simulink model "mini_project_2"  (R2024b)
settings: Solver=VariableStepAuto  StartTime=0.0  StopTime=10.0  RelTol=1e-3
values from neighbouring files (symbols this model uses):
  g = 9.81    [mini_project_2_par.m]    (also in mini_project_par.m = 9.82)
  Ic = diag([ 2 ; 2 ; 4 ])    [mini_project_2_par.m]
  m = 4    [mini_project_2_par.m]    (also in mini_project_par.m = 0.725)
  M_RB = [ m*eye(3) , zeros(3) ; zeros(3) , Ic ]    [mini_project_2_par.m]
  omega_pars = [omega_min, omega_max]    [mini_project_par.m]
  params = [m, g, h L, Ct, Ixx, Iyy, Izz]    [mini_project_par.m]
libraries: slpidlib x12, simulink_extras x7, aerolibutil x2, vrlib x1
(part 2 of 2)

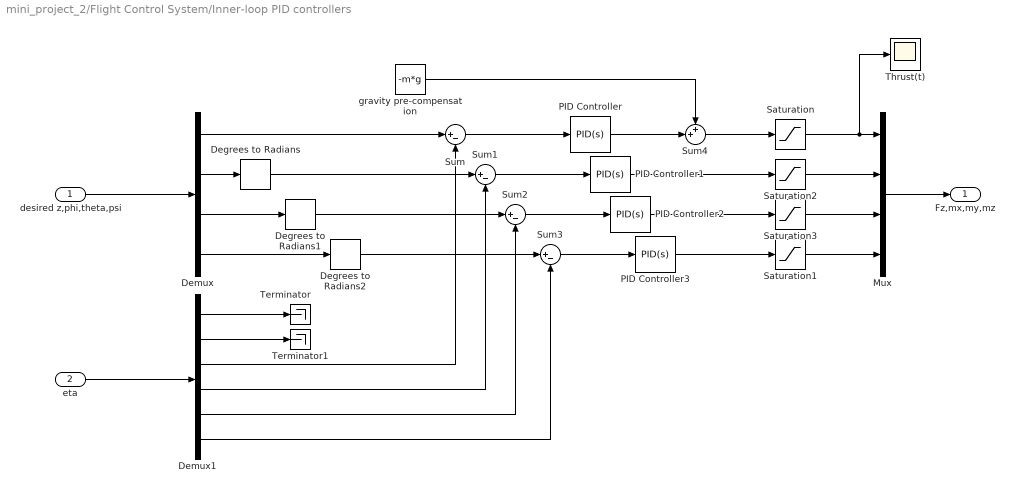
== system mini_project_2/Flight Control System/Inner-loop PID controllers ==
  desired z,phi,theta,psi : Inport
  eta : Inport  Port=2
  Degrees to Radians : simulink_extras/Transformations/Degrees to Radians
  Degrees to Radians1 : simulink_extras/Transformations/Degrees to Radians
  Degrees to Radians2 : simulink_extras/Transformations/Degrees to Radians
  Demux : Demux
  Demux1 : Demux  Outputs=6
  Mux : Mux
  PID Controller : slpidlib/PID Controller  Controller=PID  Form=Parallel  TimeDomain=Continuous-time  UseExternalTs=off  SampleTime=-1  IntegratorMethod=Forward Euler  FilterMethod=Forward Euler  ControllerParametersSource=internal  P=10  I=0  UseKiTs=off  D=20  UseExternalDerivativeSource=off  N=110  UseFilter=on  TunerSelectOption=Transfer Function Based (PID Tuner App)  InitialConditionSource=internal  InitialConditionForIntegrator=0  InitialConditionForFilter=0  DifferentiatorICPrevScaledInput=0  ExternalReset=none  TrackingMode=off  Kt=1  LimitOutput=off  SatLimitsSource=internal  UpperSaturationLimit=100  LowerSaturationLimit=-100  LinearizeAsGain=on  AntiWindupMode=none  Kb=1  LimitIntegrator=off  UpperIntegratorSaturationLimit=inf  LowerIntegratorSaturationLimit=-inf  POutMin=[]  POutMax=[]  IOutMin=[]  IOutMax=[]  DOutMin=[]  DOutMax=[]  NOutMin=[]  NOutMax=[]  SumOutMin=[]  SumOutMax=[]  SaturationOutMin=[]  SaturationOutMax=[]  PParamMin=[]  PParamMax=[]  IParamMin=[]  IParamMax=[]  DParamMin=[]  DParamMax=[]  NParamMin=[]  NParamMax=[]  KbParamMin=[]  KbParamMax=[]  KtParamMin=[]  KtParamMax=[]  KbOutMin=[]  KbOutMax=[]  KtOutMin=[]  KtOutMax=[]  IntegratorOutMin=[]  IntegratorOutMax=[]  FilterOutMin=[]  FilterOutMax=[]  SumI1OutMin=[]  SumI1OutMax=[]  SumI2OutMin=[]  SumI2OutMax=[]  SumI3OutMin=[]  SumI3OutMax=[]  SumI4OutMin=[]  SumI4OutMax=[]  SumDOutMin=[]  SumDOutMax=[]  DifferentiatorOutMin=[]  DifferentiatorOutMax=[]  FilterDiffOutCoefMin=[]  FilterDiffOutCoefMax=[]  ReciprocalOutMin=[]  ReciprocalOutMax=[]  SumDenOutMin=[]  SumDenOutMax=[]  SumNumOutMin=[]  SumNumOutMax=[]  DivideOutMin=[]  DivideOutMax=[]  UdiffTsProdOutMin=[]  UdiffTsProdOutMax=[]  NTsProdOutMin=[]  NTsProdOutMax=[]  UintegralTsProdOutMin=[]  UintegralTsProdOutMax=[]  UngainTsProdOutMin=[]  UngainTsProdOutMax=[]  ClampingZeroOutDataTypeStr=Inherit: Inherit via back propagation  ClampingZeroOutMin=[]  ClampingZeroOutMax=[]  FilterDenConstantOutDataTypeStr=Inherit: Inherit via back propagation  FilterDenConstantOutMin=[]  FilterDenConstantOutMax=[]  PCopyOutDataTypeStr=Inherit: Inherit via back propagation  PCopyOutMin=[]  PCopyOutMax=[]  NCopyOutDataTypeStr=Inherit: Inherit via back propagation  NCopyOutMin=[]  NCopyOutMax=[]  IntegratorContinuousStateAttributes=''  IntegratorStateMustResolveToSignalObject=off  IntegratorRTWStateStorageClass=Auto  FilterContinuousStateAttributes=''  FilterStateMustResolveToSignalObject=off  FilterRTWStateStorageClass=Auto  ParallelPVariant=InternalParameters  IdealPVariant=Disabled  IVariant=InternalParameters  DVariant=InternalParameters  IntegratorVariant=Continuous  SatVariant=Disabled  AWVariant=Passthrough  PCopyVariant=Disabled  TRVariant=Disabled  FdbkBlocksVariant=Forward  IdealPFdbkVariant=Disabled  SatFdbkVariant=Disabled  DerivativeFilterVariant=ContFilter  NVariant=InternalParameters  NCopyVariant=Disabled  FilterICVariant=InternalICsFilter  IntegratorICVariant=InternalICs  ExternalResetVariant=Disabled  TRSumVariant=Passthrough  SumFdbkVariant=Disabled  SumVariant=Sum_PID  TsampFilterVariant=InternalTs  TsampNgainVariant=Passthrough  TsampIntegralVariant=Disabled_SignalSpec  ExternalSaturationOutDataTypeStr=Inherit: Same as second input  DerivativeSourceVariant=ErrorSignal  PreIntVariant=InternalPreInt
  PID Controller1 : slpidlib/PID Controller  Controller=PID  Form=Parallel  TimeDomain=Continuous-time  UseExternalTs=off  SampleTime=-1  IntegratorMethod=Forward Euler  FilterMethod=Forward Euler  ControllerParametersSource=internal  P=10  I=0  UseKiTs=off  D=20  UseExternalDerivativeSource=off  N=100  UseFilter=on  TunerSelectOption=Transfer Function Based (PID Tuner App)  InitialConditionSource=internal  InitialConditionForIntegrator=0  InitialConditionForFilter=0  DifferentiatorICPrevScaledInput=0  ExternalReset=none  TrackingMode=off  Kt=1  LimitOutput=off  SatLimitsSource=internal  UpperSaturationLimit=inf  LowerSaturationLimit=-inf  LinearizeAsGain=on  AntiWindupMode=none  Kb=1  LimitIntegrator=off  UpperIntegratorSaturationLimit=inf  LowerIntegratorSaturationLimit=-inf  POutMin=[]  POutMax=[]  IOutMin=[]  IOutMax=[]  DOutMin=[]  DOutMax=[]  NOutMin=[]  NOutMax=[]  SumOutMin=[]  SumOutMax=[]  SaturationOutMin=[]  SaturationOutMax=[]  PParamMin=[]  PParamMax=[]  IParamMin=[]  IParamMax=[]  DParamMin=[]  DParamMax=[]  NParamMin=[]  NParamMax=[]  KbParamMin=[]  KbParamMax=[]  KtParamMin=[]  KtParamMax=[]  KbOutMin=[]  KbOutMax=[]  KtOutMin=[]  KtOutMax=[]  IntegratorOutMin=[]  IntegratorOutMax=[]  FilterOutMin=[]  FilterOutMax=[]  SumI1OutMin=[]  SumI1OutMax=[]  SumI2OutMin=[]  SumI2OutMax=[]  SumI3OutMin=[]  SumI3OutMax=[]  SumI4OutMin=[]  SumI4OutMax=[]  SumDOutMin=[]  SumDOutMax=[]  DifferentiatorOutMin=[]  DifferentiatorOutMax=[]  FilterDiffOutCoefMin=[]  FilterDiffOutCoefMax=[]  ReciprocalOutMin=[]  ReciprocalOutMax=[]  SumDenOutMin=[]  SumDenOutMax=[]  SumNumOutMin=[]  SumNumOutMax=[]  DivideOutMin=[]  DivideOutMax=[]  UdiffTsProdOutMin=[]  UdiffTsProdOutMax=[]  NTsProdOutMin=[]  NTsProdOutMax=[]  UintegralTsProdOutMin=[]  UintegralTsProdOutMax=[]  UngainTsProdOutMin=[]  UngainTsProdOutMax=[]  ClampingZeroOutDataTypeStr=Inherit: Inherit via back propagation  ClampingZeroOutMin=[]  ClampingZeroOutMax=[]  FilterDenConstantOutDataTypeStr=Inherit: Inherit via back propagation  FilterDenConstantOutMin=[]  FilterDenConstantOutMax=[]  PCopyOutDataTypeStr=Inherit: Inherit via back propagation  PCopyOutMin=[]  PCopyOutMax=[]  NCopyOutDataTypeStr=Inherit: Inherit via back propagation  NCopyOutMin=[]  NCopyOutMax=[]  IntegratorContinuousStateAttributes=''  IntegratorStateMustResolveToSignalObject=off  IntegratorRTWStateStorageClass=Auto  FilterContinuousStateAttributes=''  FilterStateMustResolveToSignalObject=off  FilterRTWStateStorageClass=Auto  ParallelPVariant=InternalParameters  IdealPVariant=Disabled  IVariant=InternalParameters  DVariant=InternalParameters  IntegratorVariant=Continuous  SatVariant=Disabled  AWVariant=Passthrough  PCopyVariant=Disabled  TRVariant=Disabled  FdbkBlocksVariant=Forward  IdealPFdbkVariant=Disabled  SatFdbkVariant=Disabled  DerivativeFilterVariant=ContFilter  NVariant=InternalParameters  NCopyVariant=Disabled  FilterICVariant=InternalICsFilter  IntegratorICVariant=InternalICs  ExternalResetVariant=Disabled  TRSumVariant=Passthrough  SumFdbkVariant=Disabled  SumVariant=Sum_PID  TsampFilterVariant=InternalTs  TsampNgainVariant=Passthrough  TsampIntegralVariant=Disabled_SignalSpec  ExternalSaturationOutDataTypeStr=Inherit: Same as second input  DerivativeSourceVariant=ErrorSignal  PreIntVariant=InternalPreInt
  PID Controller2 : slpidlib/PID Controller  Controller=PID  Form=Parallel  TimeDomain=Continuous-time  UseExternalTs=off  SampleTime=-1  IntegratorMethod=Forward Euler  FilterMethod=Forward Euler  ControllerParametersSource=internal  P=10  I=0  UseKiTs=off  D=20  UseExternalDerivativeSource=off  N=100  UseFilter=on  TunerSelectOption=Transfer Function Based (PID Tuner App)  InitialConditionSource=internal  InitialConditionForIntegrator=0  InitialConditionForFilter=0  DifferentiatorICPrevScaledInput=0  ExternalReset=none  TrackingMode=off  Kt=1  LimitOutput=off  SatLimitsSource=internal  UpperSaturationLimit=inf  LowerSaturationLimit=-inf  LinearizeAsGain=on  AntiWindupMode=none  Kb=1  LimitIntegrator=off  UpperIntegratorSaturationLimit=inf  LowerIntegratorSaturationLimit=-inf  POutMin=[]  POutMax=[]  IOutMin=[]  IOutMax=[]  DOutMin=[]  DOutMax=[]  NOutMin=[]  NOutMax=[]  SumOutMin=[]  SumOutMax=[]  SaturationOutMin=[]  SaturationOutMax=[]  PParamMin=[]  PParamMax=[]  IParamMin=[]  IParamMax=[]  DParamMin=[]  DParamMax=[]  NParamMin=[]  NParamMax=[]  KbParamMin=[]  KbParamMax=[]  KtParamMin=[]  KtParamMax=[]  KbOutMin=[]  KbOutMax=[]  KtOutMin=[]  KtOutMax=[]  IntegratorOutMin=[]  IntegratorOutMax=[]  FilterOutMin=[]  FilterOutMax=[]  SumI1OutMin=[]  SumI1OutMax=[]  SumI2OutMin=[]  SumI2OutMax=[]  SumI3OutMin=[]  SumI3OutMax=[]  SumI4OutMin=[]  SumI4OutMax=[]  SumDOutMin=[]  SumDOutMax=[]  DifferentiatorOutMin=[]  DifferentiatorOutMax=[]  FilterDiffOutCoefMin=[]  FilterDiffOutCoefMax=[]  ReciprocalOutMin=[]  ReciprocalOutMax=[]  SumDenOutMin=[]  SumDenOutMax=[]  SumNumOutMin=[]  SumNumOutMax=[]  DivideOutMin=[]  DivideOutMax=[]  UdiffTsProdOutMin=[]  UdiffTsProdOutMax=[]  NTsProdOutMin=[]  NTsProdOutMax=[]  UintegralTsProdOutMin=[]  UintegralTsProdOutMax=[]  UngainTsProdOutMin=[]  UngainTsProdOutMax=[]  ClampingZeroOutDataTypeStr=Inherit: Inherit via back propagation  ClampingZeroOutMin=[]  ClampingZeroOutMax=[]  FilterDenConstantOutDataTypeStr=Inherit: Inherit via back propagation  FilterDenConstantOutMin=[]  FilterDenConstantOutMax=[]  PCopyOutDataTypeStr=Inherit: Inherit via back propagation  PCopyOutMin=[]  PCopyOutMax=[]  NCopyOutDataTypeStr=Inherit: Inherit via back propagation  NCopyOutMin=[]  NCopyOutMax=[]  IntegratorContinuousStateAttributes=''  IntegratorStateMustResolveToSignalObject=off  IntegratorRTWStateStorageClass=Auto  FilterContinuousStateAttributes=''  FilterStateMustResolveToSignalObject=off  FilterRTWStateStorageClass=Auto  ParallelPVariant=InternalParameters  IdealPVariant=Disabled  IVariant=InternalParameters  DVariant=InternalParameters  IntegratorVariant=Continuous  SatVariant=Disabled  AWVariant=Passthrough  PCopyVariant=Disabled  TRVariant=Disabled  FdbkBlocksVariant=Forward  IdealPFdbkVariant=Disabled  SatFdbkVariant=Disabled  DerivativeFilterVariant=ContFilter  NVariant=InternalParameters  NCopyVariant=Disabled  FilterICVariant=InternalICsFilter  IntegratorICVariant=InternalICs  ExternalResetVariant=Disabled  TRSumVariant=Passthrough  SumFdbkVariant=Disabled  SumVariant=Sum_PID  TsampFilterVariant=InternalTs  TsampNgainVariant=Passthrough  TsampIntegralVariant=Disabled_SignalSpec  ExternalSaturationOutDataTypeStr=Inherit: Same as second input  DerivativeSourceVariant=ErrorSignal  PreIntVariant=InternalPreInt
  PID Controller3 : slpidlib/PID Controller  Controller=PID  Form=Parallel  TimeDomain=Continuous-time  UseExternalTs=off  SampleTime=-1  IntegratorMethod=Forward Euler  FilterMethod=Forward Euler  ControllerParametersSource=internal  P=10  I=0  UseKiTs=off  D=20  UseExternalDerivativeSource=off  N=100  UseFilter=on  TunerSelectOption=Transfer Function Based (PID Tuner App)  InitialConditionSource=internal  InitialConditionForIntegrator=0  InitialConditionForFilter=0  DifferentiatorICPrevScaledInput=0  ExternalReset=none  TrackingMode=off  Kt=1  LimitOutput=off  SatLimitsSource=internal  UpperSaturationLimit=inf  LowerSaturationLimit=-inf  LinearizeAsGain=on  AntiWindupMode=none  Kb=1  LimitIntegrator=off  UpperIntegratorSaturationLimit=inf  LowerIntegratorSaturationLimit=-inf  POutMin=[]  POutMax=[]  IOutMin=[]  IOutMax=[]  DOutMin=[]  DOutMax=[]  NOutMin=[]  NOutMax=[]  SumOutMin=[]  SumOutMax=[]  SaturationOutMin=[]  SaturationOutMax=[]  PParamMin=[]  PParamMax=[]  IParamMin=[]  IParamMax=[]  DParamMin=[]  DParamMax=[]  NParamMin=[]  NParamMax=[]  KbParamMin=[]  KbParamMax=[]  KtParamMin=[]  KtParamMax=[]  KbOutMin=[]  KbOutMax=[]  KtOutMin=[]  KtOutMax=[]  IntegratorOutMin=[]  IntegratorOutMax=[]  FilterOutMin=[]  FilterOutMax=[]  SumI1OutMin=[]  SumI1OutMax=[]  SumI2OutMin=[]  SumI2OutMax=[]  SumI3OutMin=[]  SumI3OutMax=[]  SumI4OutMin=[]  SumI4OutMax=[]  SumDOutMin=[]  SumDOutMax=[]  DifferentiatorOutMin=[]  DifferentiatorOutMax=[]  FilterDiffOutCoefMin=[]  FilterDiffOutCoefMax=[]  ReciprocalOutMin=[]  ReciprocalOutMax=[]  SumDenOutMin=[]  SumDenOutMax=[]  SumNumOutMin=[]  SumNumOutMax=[]  DivideOutMin=[]  DivideOutMax=[]  UdiffTsProdOutMin=[]  UdiffTsProdOutMax=[]  NTsProdOutMin=[]  NTsProdOutMax=[]  UintegralTsProdOutMin=[]  UintegralTsProdOutMax=[]  UngainTsProdOutMin=[]  UngainTsProdOutMax=[]  ClampingZeroOutDataTypeStr=Inherit: Inherit via back propagation  ClampingZeroOutMin=[]  ClampingZeroOutMax=[]  FilterDenConstantOutDataTypeStr=Inherit: Inherit via back propagation  FilterDenConstantOutMin=[]  FilterDenConstantOutMax=[]  PCopyOutDataTypeStr=Inherit: Inherit via back propagation  PCopyOutMin=[]  PCopyOutMax=[]  NCopyOutDataTypeStr=Inherit: Inherit via back propagation  NCopyOutMin=[]  NCopyOutMax=[]  IntegratorContinuousStateAttributes=''  IntegratorStateMustResolveToSignalObject=off  IntegratorRTWStateStorageClass=Auto  FilterContinuousStateAttributes=''  FilterStateMustResolveToSignalObject=off  FilterRTWStateStorageClass=Auto  ParallelPVariant=InternalParameters  IdealPVariant=Disabled  IVariant=InternalParameters  DVariant=InternalParameters  IntegratorVariant=Continuous  SatVariant=Disabled  AWVariant=Passthrough  PCopyVariant=Disabled  TRVariant=Disabled  FdbkBlocksVariant=Forward  IdealPFdbkVariant=Disabled  SatFdbkVariant=Disabled  DerivativeFilterVariant=ContFilter  NVariant=InternalParameters  NCopyVariant=Disabled  FilterICVariant=InternalICsFilter  IntegratorICVariant=InternalICs  ExternalResetVariant=Disabled  TRSumVariant=Passthrough  SumFdbkVariant=Disabled  SumVariant=Sum_PID  TsampFilterVariant=InternalTs  TsampNgainVariant=Passthrough  TsampIntegralVariant=Disabled_SignalSpec  ExternalSaturationOutDataTypeStr=Inherit: Same as second input  DerivativeSourceVariant=ErrorSignal  PreIntVariant=InternalPreInt
  Saturation{,1..3} (4 alike) : Saturate  UpperLimit=100  LowerLimit=-100
  Sum{,1..3} (4 alike) : Sum  Inputs=|+-
  Sum4 : Sum  Inputs=++|
  Terminator : Terminator
  Terminator1 : Terminator
  Thrust(t) : Scope
  gravity pre-compensation : Constant  Value=-m*g
  Fz,mx,my,mz : Outport
  wires:
  Mux/1 -> Fz,mx,my,mz/1
  Sum/1 -> PID Controller/1
  Sum1/1 -> PID Controller1/1
  PID Controller1/1 -> Saturation2/1
  PID Controller2/1 -> Saturation3/1
  PID Controller3/1 -> Saturation1/1
  Sum2/1 -> PID Controller2/1
  Sum3/1 -> PID Controller3/1
  Demux/2 -> Degrees to Radians/1
  Demux/3 -> Degrees to Radians1/1
  Demux/4 -> Degrees to Radians2/1
  desired z,phi,theta,psi/1 -> Demux/1
  eta/1 -> Demux1/1
  Demux1/1 -> Terminator/1
  Demux1/2 -> Terminator1/1
  Demux1/3 -> Sum/2
  Demux1/4 -> Sum1/2
  Demux1/5 -> Sum2/2
  Demux1/6 -> Sum3/2
  Degrees to Radians/1 -> Sum1/1
  Degrees to Radians1/1 -> Sum2/1
  Degrees to Radians2/1 -> Sum3/1
  Demux/1 -> Sum/1
  Saturation/1 -> Thrust(t)/1, Mux/1
  Saturation1/1 -> Mux/4
  Saturation2/1 -> Mux/2
  Saturation3/1 -> Mux/3
  Sum4/1 -> Saturation/1
  PID Controller/1 -> Sum4/2
  gravity pre-compensation/1 -> Sum4/1

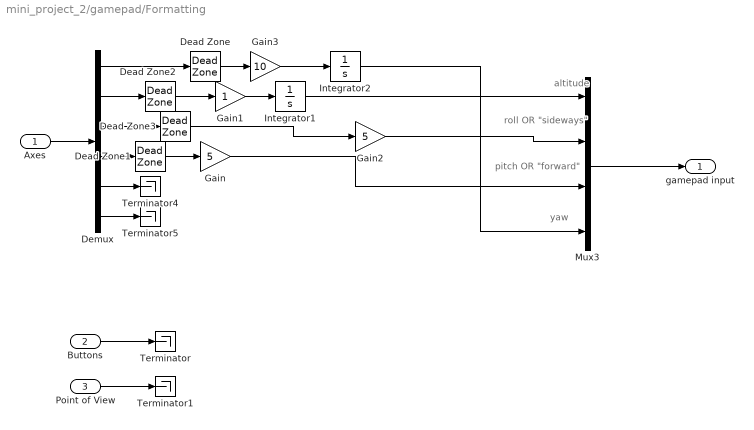
== system mini_project_2/gamepad/Formatting ==
  note: roll OR "sideways"
  note: altitude
  note: pitch OR "forward"
  note: yaw
  Axes : Inport
  Buttons : Inport  Port=2
  Point of View : Inport  Port=3
  Dead Zone{,1..3} (4 alike) : DeadZone  LowerValue=-0.2  UpperValue=0.2
  Demux : Demux  Outputs=6
  Gain : Gain  Gain=5
  Gain1 : Gain
  Gain2 : Gain  Gain=5
  Gain3 : Gain  Gain=10
  Integrator1 : Integrator  InitialCondition=-17
  Integrator2 : Integrator  InitialCondition=-45
  Mux3 : Mux
  Terminator{,1,4..5} (4 alike) : Terminator
  gamepad input : Outport
  wires:
  Mux3/1 -> gamepad input/1
  Buttons/1 -> Terminator/1
  Axes/1 -> Demux/1
  Demux/3 -> Dead Zone3/1
  Demux/5 -> Terminator4/1
  Demux/6 -> Terminator5/1
  Demux/4 -> Dead Zone1/1
  Demux/1 -> Dead Zone/1
  Dead Zone1/1 -> Gain/1
  Demux/2 -> Dead Zone2/1
  Dead Zone2/1 -> Gain1/1
  Integrator1/1 -> Mux3/1
  Dead Zone/1 -> Gain3/1
  Integrator2/1 -> Mux3/4
  Dead Zone3/1 -> Gain2/1
  Point of View/1 -> Terminator1/1
  Gain1/1 -> Integrator1/1
  Gain2/1 -> Mux3/2
  Gain/1 -> Mux3/3
  Gain3/1 -> Integrator2/1

== matlab function mini_project_2/MATLAB Function ==
  data: tau_desired_body input; T1_des output; T2_des output; delta1_des output; delta2_des output; T_desired_body input
function [T1_des, T2_des, delta1_des, delta2_des]= motor_mixer(tau_desired_body, T_desired_body)
D = 0.1;
L = 0.05;

tau_xd = tau_desired_body(1);
tau_yd = tau_desired_body(2);
tau_zd = tau_desired_body(3);
Td = T_desired_body;

delta1_des = atan2((L * tau_xd + D * tau_zd),(D * L * Td + D * tau_yd));
delta2_des = atan2((L * tau_xd - D * tau_zd),(D * L * Td - D * tau_yd));

T1_des = 1/2 * sqrt((tau_xd / D + tau_zd / L)^2 + (Td + tau_yd / L)^2);
T2_des = 1/2 * sqrt((tau_xd / D - tau_zd / L)^2 + (Td - tau_yd / L)^2);
end

== matlab function mini_project_2/Kinetic Model ==
  data: params input; Xdd output; Xd input; X input; omega input; zeta input
function Xdd = fcn(params, Xd, X, omega, zeta)
    m = params(1);
    g = params(2);
    h = params(3);
    L = params(4);
    Ct = params(5);
    Ixx = params(6);
    Iyy = params(7);
    Izz = params(8);

    x = X(1);
    xd = Xd(1);
    
    y = X(2);
    yd = Xd(2);

    z = X(3);
    zd = Xd(3);
   
    phi = X(4);
    phid = Xd(4);

    theta = X(5);
    thetad = Xd(5);

    psi = X(6);
    psid = Xd(6);

    omegaL = omega(1);
    omegaR = omega(2);

    zetaL = zeta(1);
    zetaR = zeta(2);

    u1 = Ct * (omegaR^2 * cos(zetaR) + omegaL^2 * cos(zetaL));
    u2 = Ct * (omegaR^2 * cos(zetaR) - omegaL^2 * cos(zetaL));
    u3 = Ct * (omegaR^2 * sin(zetaR) + omegaL^2 * sin(zetaL));
    u4 = Ct * (omegaR^2 * sin(zetaR) - omegaL^2 * sin(zetaL));
    
    
    xdd = - (1 / m) * (sin(phi) * sin(psi) + cos(phi) * sin(theta) * cos(psi)) * u1 - ((cos(theta) * cos(psi)) / m) * u3;
    ydd = - (1 / m) * (-sin(phi) * cos(psi) + cos(phi) * sin(theta) * sin(psi)) * u1 + ((cos(theta) * sin(psi)) / m) * u3;
    zdd = g - (1 / m) * cos(phi) * cos(theta) * u1 - (sin(theta) / m) * u3;
    phidd = (L / Ixx) * u2;
    thetadd = (h / Iyy) * u3;
    psidd = (L / Izz) * u4;


Xdd = [xdd, ydd, zdd, phidd, thetadd, psidd]';

== matlab function mini_project_2/Bicopter model/Kinematics/Kinematics ==
  data: R_be output; nu input; eta input; eta_dot output
function [R_be,eta_dot] = J_Theta(nu,eta)

% Euler angle extraction
phi = eta(4);
theta = eta(5);
psi = eta(6);

R_xphi = [ 1 0 0 ; 0 cos(phi) -sin(phi) ; 0 sin(phi) cos(phi) ];
R_ytheta = [ cos(theta) 0 sin(theta) ; 0 1 0 ; -sin(theta) 0 cos(theta) ];
R_zpsi = [ cos(psi) -sin(psi) 0 ; sin(psi) cos(psi) 0 ; 0 0 1 ];

% rotation matrix
R_be = R_zpsi * R_ytheta * R_xphi;

% angular velocity transformation
T_Theta = [ 1 sin(phi)*tan(theta) cos(phi)*tan(theta) ; 0 cos(phi) -sin(phi) ; 0 sin(phi)/cos(theta) cos(phi)/cos(theta) ];

J_Theta = [ R_be , zeros(3) ; zeros(3) , T_Theta ];

eta_dot = J_Theta*nu;

== matlab function mini_project_2/Controller/MATLAB Function2 ==
  data: u input; sat output; u_lim input; out output
function [sat, out] = saturator(u, u_lim)
out = u;
sat = 1;
u_min = u_lim(1);
u_max = u_lim(2);

if u > u_max
    out = u_max;
    sat = 0;
elseif u < u_min
    out = u_min;
    sat = 0;
end

== matlab function mini_project_2/Bicopter model/Rigid-body dynamics/Coriolis term ==
  data: nu input; Cnunu output; m input; Ic input
function Cnunu = fcn(nu,m,Ic)

v = nu(1:3);  % linear velocities (expressed in the body frame)
omega = nu(4:6); % angular velocities (expressed in the body frame)


Cnunu = [ cross(omega,m*v) ; -cross(Ic*omega,omega) ];

== matlab function mini_project_2/MATLAB Function1 ==
  data: T1 input; f_b output; tau_b output; T2 input; delta1 input; delta2 input
function [f_b, tau_b]= motor_mixer_num2(T1, T2, delta1, delta2)
D = 0.1;
L = 0.05;

A = [0, 1, 0, 1;
     D, 0, D, 0;
     0, L, 0, -L;
     L, 0, -L, 0;];

b = [T1*sin(delta1);
     T1*cos(delta1);
     T2*sin(delta2);
     T2*cos(delta2);];

res = A * b;

f_b = [0;
       0;
       res(1);];

tau_b = res(2:4);
end

== matlab function mini_project_2/MATLAB Function2 ==
  data: eul input; q output
function q = euler2quat(eul) %eul has to be [yaw pitch roll]
    q = eul2quat(eul', "ZYX");
end

== matlab function mini_project_2/MATLAB Function3 ==
  data: eta input; q output
function q = euler2quat(eta) %eul has to be [yaw pitch roll]
    roll = eta(4);
    pitch = eta(5);
    yaw = eta(6);
    eul = [yaw; pitch; roll];
    q = eul2quat(eul', "ZYX");
end

== matlab function mini_project_2/MATLAB Function4 ==
  data: qe input; omegabd output; gain input
function omegabd = get_desired_angular_velocity(qe,gain)
    nue = qe(1);
    ee = qe(2:4);

    ee = reshape(ee, 1, 3); 
    
    phi = 2 * atan2(norm(ee), nue);
    omegabd = zeros(1, 3);
     
    % Avoid division by zero if phi is very small
    if abs(sin(phi / 2)) > 1e-6
        omegabd = gain * sign(nue) * (phi / sin(phi / 2)) * ee;
    end
end

== matlab function mini_project_2/MATLAB Function5 ==
  data: ad input; y output; m input; eul input
function y = get_force(ad, m, eul)


y = u;
